simulink model "Diode_Bridge"  (R2018a)
settings: Solver=VariableStepAuto  StartTime=0.0  StopTime=10.0  RelTol=1e-3
libraries: pe_lib x4, fl_lib x3, nesl_utility x3, elec_lib x1
settings Model: Creator=Jayef  LastModifiedBy=Jayef

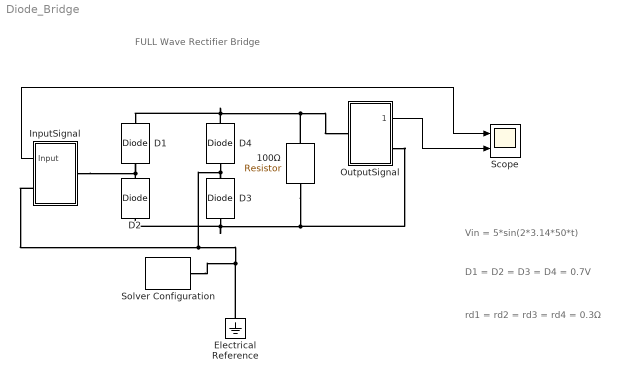
== system Diode_Bridge ==
  note: rd1 = rd2 = rd3 = rd4 = 0.3Ω
  note: D1 = D2 = D3 = D4 = 0.7V
  note: Vin = 5*sin(2*3.14*50*t)
  note: FULL Wave Rectifier Bridge
  100Ω : elec_lib/Passive Devices/Resistor  R=100 Ohm  R_tol=5  enable_R_tol=0  tol_distribution=1  nSigma=4  enable_operating_limits=0  operating_limit_action=2  max_working_voltage=100 V  power_rating=1 W  enable_faults=0  fault_action=1  R_faulted=inf Ohm  enable_temporal_fault=0  t_fault=1 s  enable_behavioral_fault=0  max_permissible_current=1 A  t_fail_on_current=1 s  noise_mode=0  sample_time=1e-3 s  repeatability=1  auto_seed=1283402414  user_seed=0  Tdevice=25 degC  alpha=3.93e-3 1/K  Tmeas=25 degC  thermal_mass=100 J/K  power_derating_T1=70 degC  power_derating_T2=155 degC  operating_temperature_range_vec=[-50, 150] degC  temperature_specify=off  temperature_priority=High  temperature=298.15 K  temperature_nominal_specify=off  temperature_nominal_unit=K  temperature_nominal_value=1
  D{1..4} (4 alike) : pe_lib/Semiconductors/Fundamental Components/Diode  Vf=0.7 V  Ron=0.3 Ohm  Goff=1e-5 1/Ohm  N_series=1  N_parallel=1  Vf_equiv=0.8 V  Ron_equiv=0.001 Ohm  Goff_equiv=1e-5 1/Ohm
      settings: SourceProductName=Simscape Power Systems  SourceProductBaseCode=PS
  Electrical Reference : fl_lib/Electrical/Electrical Elements/Electrical Reference
  InputSignal : Subsystem
  OutputSignal : Subsystem
  Scope : Scope  NumInputPorts=2
  Solver Configuration : nesl_utility/Solver Configuration  PhysicalDomain=network_engine_domain  SubClassName=solver  LeftPortType=input  RightPortType=generic  Tones=[]  Harmonics=[]  SimulateNoise=off  Profile=off  UseLocalSampling=off  EnableSwitchedLinearOptims=on  FrequencyDomain=off  UseCCode=off  RelTol=0.001  AbsTol=1e-06  MinStep=1e-09  ToWorkspace=off  RevertToSquareIcSolve=off  NumHomotopyIterations=100  PhasorMode=off  PhasorModeNumHarmonics=1  DoDC=off  ResidualTolerance=1e-09  UseLocalSolver=off  LocalSolverChoice=NE_BACKWARD_EULER_ADVANCER  LocalSolverSampleTime=0.001  DoFixedCost=off  MaxNonlinIter=3  MaxModeIter=2  LinearAlgebra=Sparse  EquationFormulation=NE_TIME_EF  DelaysMemoryBudget=1024  AutomaticFiltering=on  FilteringTimeConstant=0.001
  wires:
  InputSignal/1(Input) -> Scope/1
  OutputSignal/1(Output) -> Scope/2
  connections:
  D4/RConn1 -- D1/RConn1 -- 100Ω/LConn1 -- OutputSignal/LConn1
  D2/RConn1 -- InputSignal/LConn1 -- D1/LConn1
  Electrical Reference/LConn1 -- InputSignal/RConn1 -- D3/RConn1 -- D4/LConn1 -- Solver Configuration/RConn1
  D3/LConn1 -- OutputSignal/RConn1 -- 100Ω/RConn1 -- D2/LConn1

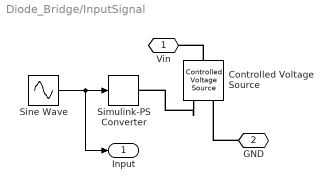
== system Diode_Bridge/InputSignal ==
  Controlled Voltage Source : fl_lib/Electrical/Electrical Sources/Controlled Voltage Source
  Simulink-PS Converter : nesl_utility/Simulink-PS Converter  PhysicalDomain=network_engine_domain  SubClassName=ps_input  LeftPortType=input  RightPortType=output  PseudoPeriodic=off  Frequencies=[]  NoiseDistribution=none  NoiseParameters=[]  Unit=1  AffineConversion=off  FilteringAndDerivatives=provide  SimscapeFilterOrder=1  InputFilterTimeConstant=0.001  UdotUserProvided=0
  Sine Wave : Sin  Amplitude=5  Frequency=2*3.14*50  SampleTime=0.00001
  Vin : PMIOPort  Side=Left
  GND : PMIOPort  Port=2  Side=Right
  Input : Outport
  wires:
  Sine Wave/1 -> Input/1, Simulink-PS Converter/1
  connections:
  Controlled Voltage Source/RConn1 -- Simulink-PS Converter/RConn1
  GND/RConn1 -- Controlled Voltage Source/RConn2
  Controlled Voltage Source/LConn1 -- Vin/RConn1

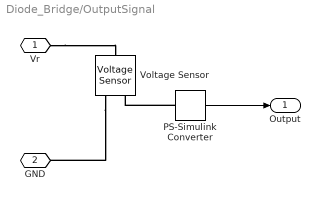
== system Diode_Bridge/OutputSignal ==
  PS-Simulink Converter : nesl_utility/PS-Simulink Converter  PhysicalDomain=network_engine_domain  SubClassName=ps_output  LeftPortType=input  RightPortType=output  PseudoPeriodic=off  Frequencies=[]  Unit=1  AffineConversion=off
  Voltage Sensor : fl_lib/Electrical/Electrical Sensors/Voltage Sensor
  Vr : PMIOPort  Side=Left
  GND : PMIOPort  Port=2  Side=Right
  Output : Outport
  wires:
  PS-Simulink Converter/1 -> Output/1
  connections:
  PS-Simulink Converter/LConn1 -- Voltage Sensor/RConn1
  Voltage Sensor/RConn2 -- GND/RConn1
  Vr/RConn1 -- Voltage Sensor/LConn1
